simulink model "Simulink_PID_LQR"  (R2025b)
settings: Solver=VariableStepAuto  StartTime=0.0  StopTime=50  RelTol=1e-3
InitFcn:
  | run("init.m");
StopFcn:
  | %run("video.m");
values from neighbouring files (symbols this model uses):
  q0_guess = [pi/3; -pi/6; pi/3]    [init.m]
  robot_params = p    [PID.m]    (also in PID_CASCATA.m)
libraries: slpidlib x1
settings Model: Creator=Acer  LastModifiedBy=Acer

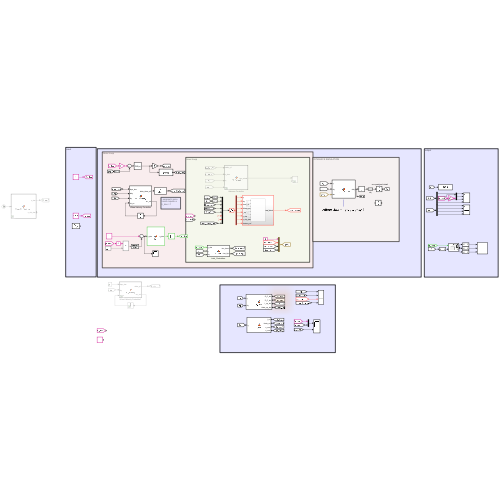
[thumbnail: Simulink's stored preview of the top-level diagram]
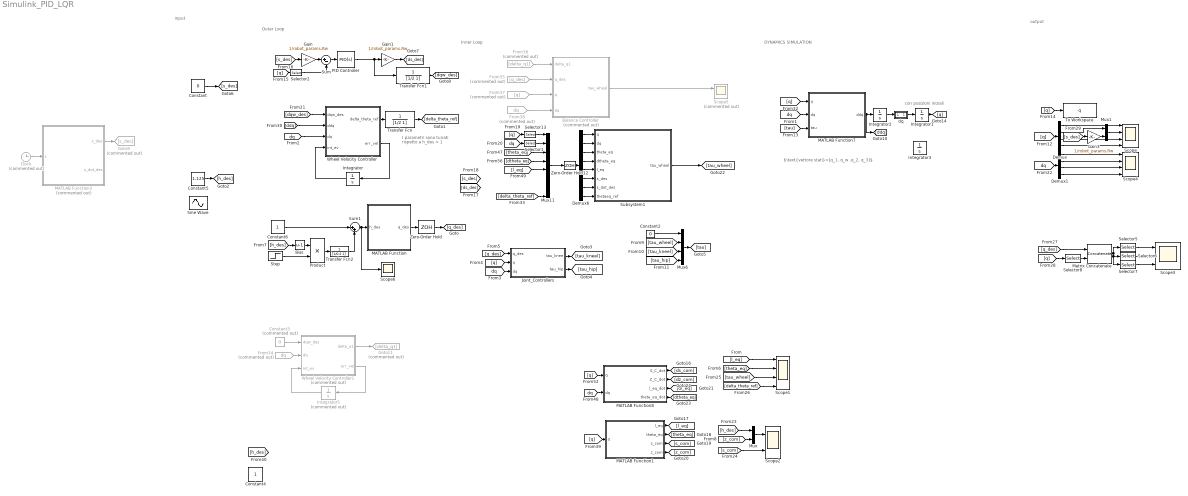
== system Simulink_PID_LQR ==
  note: I parametri sono
      | tunati rispetto a
      | h_des = 1
  note: con posizioni iniziali
  note: input
  note: output
  note: DYNAMICS SIMULATION
  note: $\text{vettore stati}=[q_1, q_w ,q_2, q_3]$
  note: Inner Loop
  note: Outer Loop
  Balance Controller : MATLAB Function  Commented=on  TreatAsAtomicUnit=on
  Bias : Bias  Bias=-1  SaturateOnIntegerOverflow=off
  Clock : Clock  Commented=on
  Constant : Constant  Value=0
  Constant2 : Constant  Value=0
  Constant3 : Constant  Commented=on  Value=0
  Constant4 : Constant
  Constant5 : Constant  Value=1.125
  Constant6 : Constant
  Demux : Demux
  Demux1 : Demux
  Demux6 : Demux  Outputs=8
  From34 : From  Commented=on  GotoTag=dq  TagVisibility=global
  From35 : From  Commented=on  GotoTag=q_des
  From36 : From  Commented=on  GotoTag=delta_q1
  From37 : From  Commented=on  GotoTag=q
  From38 : From  Commented=on  GotoTag=dq  TagVisibility=global
  Gain : Gain  Gain=1/robot_params.Rw
  Gain1 : Gain  Gain=1/robot_params.Rw
  Gain3 : Gain  Gain=1/robot_params.Rw
  Goto11 : Goto  Commented=on  GotoTag=delta_q1
  Goto9 : Goto  Commented=on  GotoTag=s_des
  Integrator : Integrator
  Integrator1 : Integrator  InitialCondition=[2.68;0;-2.34;1.23]
  Integrator2 : Integrator  InitialCondition=zeros(4,1)
  Integrator3 : Integrator  InitialCondition=[pi/2-0.1;zeros(3,1)]
  Integrator5 : Integrator  Commented=on
  Joint_Controllers : MATLAB Function  TreatAsAtomicUnit=on
  MATLAB Function : MATLAB Function  TreatAsAtomicUnit=on
  MATLAB Function1 : MATLAB Function  TreatAsAtomicUnit=on
  MATLAB Function2 : MATLAB Function  Commented=on  TreatAsAtomicUnit=on
  MATLAB Function7 : MATLAB Function  TreatAsAtomicUnit=on
  MATLAB Function8 : MATLAB Function  TreatAsAtomicUnit=on
  Matrix Concatenate : Concatenate  Mode=Multidimensional array  ConcatenateDimension=2
  Mux : Mux  Inputs=2
  Mux1 : Mux  Inputs=2
  Mux11 : Mux  Inputs=[1 1 1 1 1 1 1 1]
  Mux6 : Mux
  PID Controller : slpidlib/PID Controller  Controller=PID  Form=Parallel  TimeDomain=Continuous-time  UseExternalTs=off  SampleTime=-1  IntegratorMethod=Forward Euler  FilterMethod=Forward Euler  ControllerParametersSource=internal  P=0.0245  I=0.01  UseKiTs=off  D=0  UseExternalDerivativeSource=off  N=100  UseFilter=on  TunerSelectOption=Transfer Function Based (PID Tuner App)  InitialConditionSource=internal  InitialConditionForIntegrator=0  InitialConditionForFilter=0  DifferentiatorICPrevScaledInput=0  ExternalReset=none  TrackingMode=off  Kt=1  LimitOutput=off  SatLimitsSource=internal  UpperSaturationLimit=inf  LowerSaturationLimit=-inf  LinearizeAsGain=on  AntiWindupMode=none  Kb=1  LimitIntegrator=off  UpperIntegratorSaturationLimit=inf  LowerIntegratorSaturationLimit=-inf  POutMin=[]  POutMax=[]  IOutMin=[]  IOutMax=[]  DOutMin=[]  DOutMax=[]  NOutMin=[]  NOutMax=[]  SumOutMin=[]  SumOutMax=[]  SaturationOutMin=[]  SaturationOutMax=[]  PParamMin=[]  PParamMax=[]  IParamMin=[]  IParamMax=[]  DParamMin=[]  DParamMax=[]  NParamMin=[]  NParamMax=[]  KbParamMin=[]  KbParamMax=[]  KtParamMin=[]  KtParamMax=[]  KbOutMin=[]  KbOutMax=[]  KtOutMin=[]  KtOutMax=[]  IntegratorOutMin=[]  IntegratorOutMax=[]  FilterOutMin=[]  FilterOutMax=[]  SumI1OutMin=[]  SumI1OutMax=[]  SumI2OutMin=[]  SumI2OutMax=[]  SumI3OutMin=[]  SumI3OutMax=[]  SumI4OutMin=[]  SumI4OutMax=[]  SumDOutMin=[]  SumDOutMax=[]  DifferentiatorOutMin=[]  DifferentiatorOutMax=[]  FilterDiffOutCoefMin=[]  FilterDiffOutCoefMax=[]  ReciprocalOutMin=[]  ReciprocalOutMax=[]  SumDenOutMin=[]  SumDenOutMax=[]  SumNumOutMin=[]  SumNumOutMax=[]  DivideOutMin=[]  DivideOutMax=[]  UdiffTsProdOutMin=[]  UdiffTsProdOutMax=[]  NTsProdOutMin=[]  NTsProdOutMax=[]  UintegralTsProdOutMin=[]  UintegralTsProdOutMax=[]  UngainTsProdOutMin=[]  UngainTsProdOutMax=[]  ClampingZeroOutDataTypeStr=Inherit: Inherit via back propagation  ClampingZeroOutMin=[]  ClampingZeroOutMax=[]  FilterDenConstantOutDataTypeStr=Inherit: Inherit via back propagation  FilterDenConstantOutMin=[]  FilterDenConstantOutMax=[]  PCopyOutDataTypeStr=Inherit: Inherit via back propagation  PCopyOutMin=[]  PCopyOutMax=[]  NCopyOutDataTypeStr=Inherit: Inherit via back propagation  NCopyOutMin=[]  NCopyOutMax=[]  IntegratorContinuousStateAttributes=''  IntegratorStateMustResolveToSignalObject=off  IntegratorRTWStateStorageClass=Auto  FilterContinuousStateAttributes=''  FilterStateMustResolveToSignalObject=off  FilterRTWStateStorageClass=Auto  ParallelPVariant=InternalParameters  IdealPVariant=Disabled  IVariant=InternalParameters  DVariant=InternalParameters  IntegratorVariant=Continuous  SatVariant=Disabled  AWVariant=Passthrough  PCopyVariant=Disabled  TRVariant=Disabled  FdbkBlocksVariant=Forward  IdealPFdbkVariant=Disabled  SatFdbkVariant=Disabled  DerivativeFilterVariant=ContFilter  NVariant=InternalParameters  NCopyVariant=Disabled  FilterICVariant=InternalICsFilter  IntegratorICVariant=InternalICs  ExternalResetVariant=Disabled  TRSumVariant=Passthrough  SumFdbkVariant=Disabled  SumVariant=Sum_PID  TsampFilterVariant=InternalTs  TsampNgainVariant=Passthrough  TsampIntegralVariant=Disabled_SignalSpec  ExternalSaturationOutDataTypeStr=Inherit: Same as second input  DerivativeSourceVariant=ErrorSignal  PreIntVariant=InternalPreInt
  Product : Product
  Scope : Scope  NumInputPorts=4
      settings: ActiveDisplayString=4  Title=q3  ActiveDisplayYMinimum=0.54816022439736856  ActiveDisplayYMaximum=1.3057599750669591
  Scope1 : Scope  NumInputPorts=4
      settings: ActiveDisplayString=4  Title=Delta_theta_ref  ActiveDisplayYMinimum=-0.047873246159911287  ActiveDisplayYMaximum=0.27907655031491813
  Scope2 : Scope  NumInputPorts=2
      settings: ActiveDisplayYMinimum=0.29186136198287116  ActiveDisplayYMaximum=1.3009042931130141  DataLoggingVariableName=ScopeData2
  Scope3 : Scope  NumInputPorts=3
      settings: ActiveDisplayYMinimum=2.02772604544463  ActiveDisplayYMaximum=2.8223539236982456  DataLoggingVariableName=ScopeData3
  Scope4 : Scope  NumInputPorts=4
      settings: Title=dq1  ActiveDisplayYMinimum=-1.1906100272021516  ActiveDisplayYMaximum=1.6920979215580041  DataLoggingVariableName=ScopeData4
  Scope5 : Scope  Commented=on  NumInputPorts=2
      settings: ActiveDisplayYMinimum=-45.318412142081343  ActiveDisplayYMaximum=55.56419413732629  DataLoggingVariableName=ScopeData5
  Scope6 : Scope
      settings: ActiveDisplayYMinimum=0.98439000764646023  ActiveDisplayYMaximum=1.1404899311818584  DataLoggingVariableName=ScopeData6
  Selector1 : Selector  InputPortWidth=4  IndexOptions=Index vector (dialog)  Indices=[2]  OutputSizes=1
  Selector13 : Selector  InputPortWidth=4  IndexOptions=Index vector (dialog)  Indices=[2]  OutputSizes=1
  Selector2 : Selector  InputPortWidth=4  IndexOptions=Index vector (dialog)  Indices=[2]  OutputSizes=1
  Selector5 : Selector  NumberOfDimensions=2  InputPortWidth=3  IndexOptions=Index vector (dialog),Index vector (dialog)  Indices=[1],[1 2]  OutputSizes=1,1
  Selector6 : Selector  NumberOfDimensions=2  InputPortWidth=3  IndexOptions=Index vector (dialog),Index vector (dialog)  Indices=[2],[1 2]  OutputSizes=1,1
  Selector7 : Selector  NumberOfDimensions=2  InputPortWidth=3  IndexOptions=Index vector (dialog),Index vector (dialog)  Indices=[3],[1 2]  OutputSizes=1,1
  Selector8 : Selector  InputPortWidth=4  IndexOptions=Index vector (dialog)  Indices=[1 3 4]  OutputSizes=1
  Sine Wave : Sin  Amplitude=0.1  Bias=0.7  SampleTime=0
  Step : Step  Time=0  SampleTime=0
  Subsystem1 : Subsystem
  Sum : Sum  Inputs=|+-
  Sum1 : Sum  Inputs=|++
  To Workspace : ToWorkspace  VariableName=q  SaveFormat=Timeseries  SampleTime=-1
  Transfer Fcn : TransferFcn  Denominator=[1/2 1]
  Transfer Fcn1 : TransferFcn  Denominator=[1/2 1]
  Transfer Fcn2 : TransferFcn  Denominator=[1/0.2 1]
  Wheel Velocity Controller : MATLAB Function  TreatAsAtomicUnit=on
  Wheel Velocity Controller1 : MATLAB Function  Commented=on  TreatAsAtomicUnit=on
  Zero-Order Hold : ZeroOrderHold  SampleTime=-1
  Zero-Order Hold12 : ZeroOrderHold  SampleTime=1e-3
  dq : Subsystem
  wires:
  [tau] -> MATLAB Function7/3(tau)
  [q] -> MATLAB Function7/1(q)
  Integrator1/1 -> [q]
  MATLAB Function7/1(ddq) -> [ddq], Integrator2/1
  [dq] -> MATLAB Function7/2(dq)
  [dq] -> Wheel Velocity Controller/3(dq)
  Integrator2/1 -> dq/1(In1)
  dq/1(Out1) -> Integrator1/1
  [dq] -> Joint_Controllers/3(dq)
  [q] -> Joint_Controllers/2(q)
  Wheel Velocity Controller/2(err_vel) -> Integrator/1
  Integrator/1 -> Wheel Velocity Controller/4(int_ev)
  MATLAB Function/1(q_des) -> Zero-Order Hold/1
  [tau_wheel] -> Mux6/2
  [tau_kneel] -> Mux6/3
  [tau_hip] -> Mux6/4
  Demux/1 -> Scope/1
  Demux/3 -> Scope/3
  Demux/4 -> Scope/4
  [q] -> Demux/1
  Constant2/1 -> Mux6/1
  Mux6/1 -> [tau]
  [q] -> To Workspace/1
  Demux6/2 -> Subsystem1/2(dq)
  [dtheta_eq] -> Mux11/4
  Demux6/1 -> Subsystem1/1(q)
  [theta_eq] -> Mux11/3
  Demux6/5 -> Subsystem1/5(l_eq)
  [l_eq] -> Mux11/5
  Demux6/3 -> Subsystem1/3(theta_eq)
  Selector1/1 -> Mux11/2
  [q] -> Selector13/1
  [dq] -> Selector1/1
  Selector13/1 -> Mux11/1
  Demux6/4 -> Subsystem1/4(dtheta_eq)
  Demux6/7 -> Subsystem1/7(s_dot_des)
  Demux6/6 -> Subsystem1/6(s_des)
  MATLAB Function1/4(z_com) -> [z_com]
  MATLAB Function8/2(Z_C_dot) -> [dz_com]
  MATLAB Function1/3(s_com) -> [s_com]
  MATLAB Function8/4(theta_eq_dot) -> [dtheta_eq]
  MATLAB Function1/1(l_eq) -> [l_eq]
  [q] -> MATLAB Function8/1(q)
  [q] -> MATLAB Function1/1(q)
  MATLAB Function1/2(theta_eq) -> [theta_eq]
  MATLAB Function8/3(l_eq_dot) -> [dl_eq]
  [dq] -> MATLAB Function8/2(dq)
  MATLAB Function8/1(S_C_dot) -> [ds_com]
  [l_eq] -> Scope1/1
  [theta_eq] -> Scope1/2
  Constant5/1 -> [h_des]
  [z_com] -> Mux/2
  [h_des] -> Mux/1
  [s_com] -> Scope2/2
  Mux/1 -> Scope2/1
  [q_des] -> Matrix Concatenate/1
  Matrix Concatenate/1 -> Selector7/1, Selector6/1, Selector5/1
  Selector5/1 -> Scope3/1
  Selector6/1 -> Scope3/2
  Selector7/1 -> Scope3/3
  [q] -> Selector8/1
  Selector8/1 -> Matrix Concatenate/2
  ? -> Mux11/7
  [q_des] -> Joint_Controllers/1(q_des)
  Joint_Controllers/1(tau_knee) -> [tau_kneel]
  Joint_Controllers/2(tau_hip) -> [tau_hip]
  [tau_wheel] -> Scope1/3
  Mux11/1 -> Zero-Order Hold12/1
  Zero-Order Hold12/1 -> Demux6/1
  [delta_theta_ref] -> Scope1/4
  ? -> Mux11/6
  Zero-Order Hold/1 -> [q_des]
  [delta_theta_ref] -> Mux11/8
  Demux6/8 -> Subsystem1/8(thetaeq_ref)
  Constant/1 -> [s_des]
  [q] -> Selector2/1
  [s_des] -> Gain/1
  Gain/1 -> Sum/1
  Selector2/1 -> Sum/2
  Sum/1 -> PID Controller/1
  Gain1/1 -> [ds_des]
  Demux1/4 -> Scope4/4
  Demux1/3 -> Scope4/3
  Demux1/1 -> Scope4/1
  Demux1/2 -> Scope4/2
  [dq] -> Demux1/1
  Clock/1 -> MATLAB Function2/1(t)
  MATLAB Function2/1(s_des) -> Goto9/1
  [s_des] -> Gain3/1
  Mux1/1 -> Scope/2
  Demux/2 -> Mux1/1
  Gain3/1 -> Mux1/2
  Wheel Velocity Controller/1(delta_theta_ref) -> Transfer Fcn/1
  Transfer Fcn/1 -> [delta_theta_ref]
  [ddq] -> Wheel Velocity Controller/2(ddq)
  Transfer Fcn1/1 -> [dqw_des]
  Constant6/1 -> Sum1/1
  Sum1/1 -> Scope6/1, MATLAB Function/1(h_des)
  [dqw_des] -> Wheel Velocity Controller/1(dqw_des)
  Subsystem1/1(tau_wheel) -> [tau_wheel]
  Balance Controller/1(tau_wheel) -> Scope5/1
  From34/1 -> Wheel Velocity Controller1/2(dq)
  Constant3/1 -> Wheel Velocity Controller1/1(dqw_des)
  Wheel Velocity Controller1/2(err_vel) -> Integrator5/1
  Integrator5/1 -> Wheel Velocity Controller1/3(int_ev)
  Wheel Velocity Controller1/1(delta_q1) -> Goto11/1
  From35/1 -> Balance Controller/2(q_des)
  From36/1 -> Balance Controller/1(delta_q1)
  From38/1 -> Balance Controller/4(dq)
  From37/1 -> Balance Controller/3(q)
  [h_des] -> Bias/1
  Bias/1 -> Product/1
  Step/1 -> Product/2
  Product/1 -> Transfer Fcn2/1
  Transfer Fcn2/1 -> Sum1/2
  PID Controller/1 -> Transfer Fcn1/1, Gain1/1

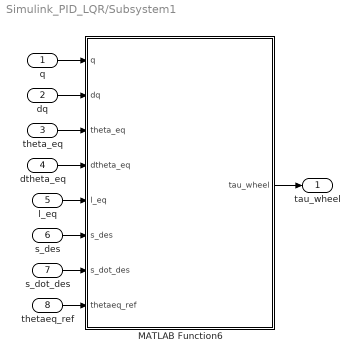
== system Simulink_PID_LQR/Subsystem1 ==
  q : Inport
  dq : Inport  Port=2
  theta_eq : Inport  Port=3
  dtheta_eq : Inport  Port=4
  l_eq : Inport  Port=5
  s_des : Inport  Port=6
  s_dot_des : Inport  Port=7
  thetaeq_ref : Inport  Port=8
  MATLAB Function6 : MATLAB Function  TreatAsAtomicUnit=on
  tau_wheel : Outport
  wires:
  dtheta_eq/1 -> MATLAB Function6/4(dtheta_eq)
  l_eq/1 -> MATLAB Function6/5(l_eq)
  s_dot_des/1 -> MATLAB Function6/7(s_dot_des)
  q/1 -> MATLAB Function6/1(q)
  theta_eq/1 -> MATLAB Function6/3(theta_eq)
  dq/1 -> MATLAB Function6/2(dq)
  s_des/1 -> MATLAB Function6/6(s_des)
  MATLAB Function6/1(tau_wheel) -> tau_wheel/1
  thetaeq_ref/1 -> MATLAB Function6/8(thetaeq_ref)

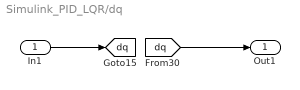
== system Simulink_PID_LQR/dq ==
  In1 : Inport
  Out1 : Outport
  tag scope: dq=global
  wires:
  In1/1 -> [dq]
  [dq] -> Out1/1

== matlab function Simulink_PID_LQR/MATLAB Function8 ==
  data: q input; dq input; S_C_dot output; Z_C_dot output; l_eq_dot output; theta_eq_dot output; robot_params parameter
function [S_C_dot, Z_C_dot, l_eq_dot, theta_eq_dot] = J_CoM(q,dq,robot_params)
    %#codegen
    % CALCOLA_VELOCITA_COM_SIMULINK Calcola le velocità del CoM e del pendolo 
    % equivalente (WIP) per l'utilizzo in Simulink.
    
    % --- 1. Estrazione Variabili di Stato ---
    q1 = q(1);
    q2 = q(3);
    q3 = q(4);
    
    % --- 2. Estrazione Parametri Robot ---
    l1 = robot_params.l1;
    l2 = robot_params.l2;
    l3 = robot_params.l3;
    
    m1 = robot_params.m1;
    m2 = robot_params.m2;
    m3 = robot_params.m3;
    m_upper = m1 + m2 + m3;
    
    % --- 3. Costanti Raggruppate per l'Analitica ---
    K1 = (m1 * (l1/2) + m2 * l1 + m3 * l1) / m_upper;
    K2 = (m2 * (l2/2) + m3 * l2) / m_upper;
    K3 = (m3 * (l3/2)) / m_upper;
    
    % --- 4. Ricalcolo Posizione CoM ---
    S_C = K1*cos(q1) + K2*cos(q1+q2) + K3*sin(q3);
    Z_C = K1*sin(q1) + K2*sin(q1+q2) + K3*cos(q3);
    
    % --- 5. Calcolo Jacobiano (J_CoM) ---
    % Preallocazione statica della matrice 2x4 per compatibilità C/C++
    J_CoM = zeros(2, 4);
    
   % --- 5. Calcolo Jacobiano (J_CoM) ---
    % Preallocazione statica della matrice 2x4 per compatibilità C/C++
    J_CoM = zeros(2, 4);
    
    % Derivate parziali di S_C (Prima Riga)
    J_CoM(1, 1) = -K1*sin(q1) - K2*sin(q1+q2); % <--- CORRETTO: indice (1,1) per dq1
    J_CoM(1, 3) = -K2*sin(q1+q2);              % <--- CORRETTO: indice (1,3) per dq2
    J_CoM(1, 4) =  K3*cos(q3);                 % <--- CORRETTO: indice (1,4) per dq3
    
    % Derivate parziali di Z_C (Seconda Riga)
    J_CoM(2, 1) =  K1*cos(q1) + K2*cos(q1+q2); % <--- CORRETTO: indice (2,1) per dq1
    J_CoM(2, 3) =  K2*cos(q1+q2);              % <--- CORRETTO: indice (2,3) per dq2
    J_CoM(2, 4) = -K3*sin(q3);                 % <--- CORRETTO: indice (2,4) per dq3
    % --- 6. Calcolo Velocità Cartesiane ---
    % V_C = [S_C_dot; Z_C_dot]
    V_C = J_CoM * dq;
    S_C_dot = V_C(1);
    Z_C_dot = V_C(2);
    
    % --- 7. Derivate del Pendolo Equivalente e Gestione Singolarità ---
    l_eq_sq = S_C^2 + Z_C^2;
    l_eq = sqrt(l_eq_sq);
    

        l_eq_dot = (S_C * S_C_dot + Z_C * Z_C_dot) / l_eq;
        theta_eq_dot = (S_C_dot * Z_C - S_C * Z_C_dot) / l_eq_sq;
   end

== matlab function Simulink_PID_LQR/MATLAB Function2 ==
  data: t input; s_des output; s_dot_des output
function [s_des, s_dot_des] = Smooth_Trajectory(t)
    % PRE-ALLOCAZIONE PER IL CODER
    s_des = 0.0;
    s_dot_des = 0.0;
    
    % PARAMETRI DELLA TRAIETTORIA
    t_start = 5.0;       % Il robot inizia a muoversi a 2 secondi
    t_end = 15.0;         % Arriva a destinazione a 5 secondi (3 secondi di viaggio)
    s_final = .5;       % Destinazione orizzontale (1 metro)
    
    % LOGICA DEL MOVIMENTO
    if t <= t_start
        % Prima di partire, resta fermo
        s_des = 0.0;
        s_dot_des = 0.0;
        
    elseif t >= t_end
        % Arrivato a destinazione, fermati
        s_des = s_final;
        s_dot_des = 0.0;
        
    else
        % FASE DI MOTO: Polinomio Cubico (Minimum Jerk Trajectory)
        % Normalizziamo il tempo tra 0 e 1 per la durata del viaggio
        tau = (t - t_start) / (t_end - t_start);
        
        % Posizione (Profilo a "S" morbida)
        s_des = s_final * (3*tau^2 - 2*tau^3);
        
        % Velocità (Derivata della posizione, forma a campana)
        s_dot_des = s_final * (6*tau - 6*tau^2) / (t_end - t_start);
    end
end

== matlab function Simulink_PID_LQR/Wheel Velocity Controller ==
  data: dqw_des input; ddq input; delta_theta_ref output; dq input; int_ev input; err_vel output
function [delta_theta_ref, err_vel] = PID_Velocity(dqw_des, ddq, dq,int_ev)
    err_vel = dqw_des - dq(2); 

    % Valori tollerabili per non saturare al primo respiro
    Kp_v = 0.06; %0.06
    
    % L'integrale ORA è vitale per compensare lo sbilanciamento di +0.16 rad
    Ki_v =0.1; %0.1; 
    Kd_v= 0.0235; %0.02
    % VIA IL SEGNO MENO!
    delta_theta_ref =(Kp_v * err_vel + Ki_v * int_ev -Kd_v*ddq(2));

    
    
    % Saturazione a 0.2 rad (circa 11 gradi) è un limite sicuro per l'LQR
    delta_theta_ref = max(min(delta_theta_ref, 0.3), -0.3); 
end

== matlab function Simulink_PID_LQR/Joint_Controllers ==
  data: q_des input; tau_knee output; q input; tau_hip output; dq input
function [tau_knee, tau_hip] = PD_Joints(q_des, q, dq)

    Kp_j = 800; 
    Kd_j = 150;  
    
    e2 = q_des(2) - q(3);
    de2 = 0 - dq(3);
    tau_knee = Kp_j * e2 + Kd_j * de2;
    
    e3 = q_des(3) - q(4);
    de3 = 0 - dq(4);
    tau_hip = Kp_j * e3 + Kd_j * de3;

== matlab function Simulink_PID_LQR/MATLAB Function ==
  settings: updateMethod=DISCRETE  sampleTime=0.1
  data: h_des input; q_des output; robot_params parameter; q0_guess parameter
function q_des = fcn(h_des, robot_params, q0_guess)
    % 1. Pre-allocazione per dire a Simulink che uscirà un vettore 3x1
    q_des = zeros(3,1);
    
    % 2. Dichiara la TUA funzione esterna come estrinseca (non fsolve)
    coder.extrinsic('calcola_target_cinematici');
    
    % 3. Inizializza la variabile temporanea per aiutare il Coder con i tipi
    q_des_calc = zeros(3,1);
    
    % 4. Richiama la funzione (il calcolo viene "appaltato" a MATLAB)
    q_des_calc = calcola_target_cinematici(h_des, robot_params, q0_guess);
    
    % 5. Assegnazione sicura all'uscita
    if ~isempty(q_des_calc)
        q_des = q_des_calc;
    end
end

== matlab function Simulink_PID_LQR/Balance Controller ==
  data: delta_q1 input; tau_wheel output; q_des input; q input; dq input
function tau_wheel = PD_Wheel(delta_q1, q_des, q, dq)

% Il target reale dello stinco è ora modificato dal loop di velocità!
    q1_target_new = q_des(1) + delta_q1; 
    
    Kp_w = 400;  % Guadagno proporzionale ruota
    Kd_w = 80;   % Guadagno derivativo ruota
    
    e1 = q1_target_new - q(1);
    de1 = 0 - dq(1);
    
    % Generazione coppia di bilanciamento
    tau_wheel = Kp_w * e1 + Kd_w * de1;

== matlab function Simulink_PID_LQR/Wheel Velocity Controller1 ==
  data: dqw_des input; delta_q1 output; dq input; int_ev input; err_vel output
function [delta_q1, err_vel] = PI_Velocity(dqw_des, dq, int_ev)

    % dqw_des velocita di riferimento della ruota
    
    err_vel = dqw_des - dq(2); % Errore di velocità della ruota
    
    % Guadagni PI (relativamente piccoli perché mappano velocità in radianti di inclinazione)
    Kp_v = 0.08; 
    Ki_v = 0.06;

    % L'output del loop di velocità è un "Angle Offset" (delta_q1)
    delta_q1 = -(Kp_v * err_vel + Ki_v * int_ev);

    % Saturazione di sicurezza per evitare che l'offset richieda inclinazioni estreme
    delta_q1 = max(min(delta_q1, 0.2), -0.2);

== matlab function Simulink_PID_LQR/MATLAB Function1 ==
  data: q input size=4; l_eq output; theta_eq output; s_com output; z_com output; robot_params parameter
function [l_eq,theta_eq, s_com, z_com] = CoM(q,robot_params)

[l_eq,theta_eq, s_com, z_com] = calcola_CoM_equivalente(q, robot_params);

end

== matlab function Simulink_PID_LQR/MATLAB Function7 ==
  data: q input; ddq output size=4; dq input; tau input
function ddq =  whole_robot_2D(q, dq, tau)
    % tau è il vettore delle coppie/forze generalizzate in ingresso (4x1)
    
    [M, CdQ, G] = calc_dynamics(q, dq);

    %% equazione del moto: M*ddq + C*dq + G = tau
    % In MATLAB/Simulink si usa l'operatore mldivide (\) per invertire M in modo robusto
    ddq = M \ (tau - CdQ - G);
end

== matlab function Simulink_PID_LQR/Subsystem1/MATLAB Function6 ==
  data: q input; tau_wheel output; dq input; theta_eq input; dtheta_eq input; l_eq input; s_des input; s_dot_des input; robot_params parameter; thetaeq_ref input
function tau_wheel  = TV_LQR_Online(q, dq, theta_eq, dtheta_eq, l_eq, s_des, s_dot_des, robot_params, thetaeq_ref)
    % Comando magico per poter usare lqr() dentro Simulink senza errori di compilazione
    coder.extrinsic('lqr');

    
    % --- PROTEZIONE DA DIVISIONE PER ZERO ---
    %l_eq = max(l_eq, 0.4); 
    
    % --- 1. Estrazione Parametri Fisici dalla Struct ---
    m_w = robot_params.mw;      
    I_w = robot_params.Iw;      
    r   = robot_params.Rw;           
    m_b = robot_params.mb; 
    g   = 9.81;
    
    % --- 2. Costruzione Stato (X) e Riferimento (X_des) ---
    % Adesso lo stato è a 4 variabili: [s; theta_eq; s_dot; theta_dot]
    s = q * r;
    s_dot = dq * r;
    X = [s; theta_eq; s_dot; dtheta_eq];
    
    X_des = [s_des; 0; s_dot_des; 0];
    
    % --- 3. Ricalcolo Dinamico Matrici A (4x4) e B (4x1) ---
    I_y = (1/3) * m_b * l_eq^2;
    
    % Denominatore adattato per UNA SOLA ruota (tolti i '2*')
    den = I_w*(I_y + m_b*l_eq^2) + (l_eq^2*m_b*m_w + I_y*(m_b + m_w)*r^2);
    
    % Coefficienti adattati per UNA SOLA ruota
    a_1 = - (g * l_eq^2 * m_b^2 * r^2) / den;
    a_2 = (g * l_eq * m_b * (I_w + (m_b + m_w)*r^2)) / den;
    b_1 = (r * (I_y + l_eq*m_b*(l_eq + r))) / den;
    b_2 = - (I_w + r*(l_eq*m_b + (m_b + m_w)*r)) / den;
    
    A = zeros(4,4);
    A(1,3) = 1; 
    A(2,4) = 1; 
    A(3,2) = a_1;
    A(4,2) = a_2;
    
    B = zeros(4,1);
    B(3,1) = b_1; 
    B(4,1) = b_2; 
    
% --- 4. Calcolo LQR Online ---
    % Rimettiamo un peso > 0 sulla posizione (es. 10) per garantire la rilevabilità
    Q = diag([0.1, 10000, .1, 10]); 
    R = 0.1;
    
    K = zeros(1, 4); 
    K = lqr(A, B, Q, R); % Ora non darà più errore!
% --- 5. Azione di Controllo (Inseguimento Traiettoria Reale) ---
    
    % ATTENZIONE ALLA CONVENZIONE:
    % Per usare u = -K * X_error, X_error DEVE essere (Stato_Attuale - Riferimento)
    % Se il robot cade in avanti, theta_eq è positivo, s_dot è positivo.
    
    X_error = [ (s - s_des);             % Errore di posizione lineare
                (theta_eq - thetaeq_ref);          % Errore di angolo (POSITIVO se cade in avanti)
                (s_dot - s_dot_des);     % Errore di velocità lineare
                (dtheta_eq - 0) ];       % Errore di velocità angolare
    
    % La matrice K compenserà l'errore con il segno corretto
    tau_wheel = -K * X_error;
end
